simulink model "questao3simlcsd2"  (R2026a)
settings: Solver=VariableStepAuto
settings Model: Creator=shumy  LastModifiedBy=shumy

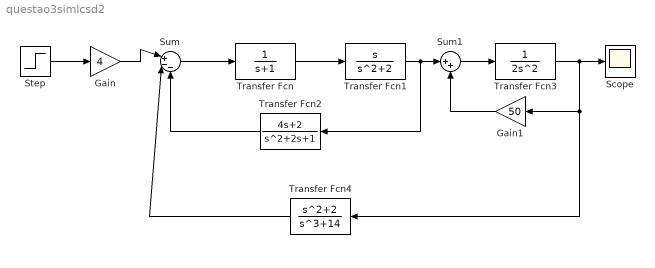
== system questao3simlcsd2 ==
  Gain : Gain  Gain=4
  Gain1 : Gain  Gain=50
  Scope : Scope
      settings: ActiveDisplayYMinimum=-5.283488255547531E+15  ActiveDisplayYMaximum=4.7551394299927792E+16
  Step : Step  SampleTime=0
  Sum : Sum  Inputs=|+--
  Sum1 : Sum  Inputs=|++
  Transfer Fcn : TransferFcn  Denominator=[1 1]
  Transfer Fcn1 : TransferFcn  Numerator=[1 0]  Denominator=[1 0 2]
  Transfer Fcn2 : TransferFcn  Numerator=[4 2]
  Transfer Fcn3 : TransferFcn  Denominator=[2 0 0]
  Transfer Fcn4 : TransferFcn  Numerator=[1 0 2]  Denominator=[1 0 0 14]
  wires:
  Step/1 -> Gain/1
  Gain/1 -> Sum/1
  Sum/1 -> Transfer Fcn/1
  Transfer Fcn/1 -> Transfer Fcn1/1
  Transfer Fcn1/1 -> Sum1/1, Transfer Fcn2/1
  Transfer Fcn2/1 -> Sum/3
  Sum1/1 -> Transfer Fcn3/1
  Transfer Fcn3/1 -> Transfer Fcn4/1, Gain1/1, Scope/1
  Gain1/1 -> Sum1/2
  Transfer Fcn4/1 -> Sum/2
